simulink model "simu1"  (R2014b)
settings: Solver=VariableStepAuto  StartTime=0.0  StopTime=10.0  RelTol=1e-3
undefined symbols (not defined in the file or in its folder): As, Gamma1
libraries: simulink_extras x1
settings Model: Creator=e1302259  LastModifiedBy=Wissale !
settings DataIOCC: LimitDataPoints=off  SaveFormat=Dataset
settings OptimizationCC: UseDivisionForNetSlopeComputation=off  SimCompilerOptimization=off
settings DebuggingCC: SolverPrmCheckMsg=none  FrameProcessingCompatibilityMsg=error
settings HardwareCC: ProdBitPerPointer=64  ProdLargestAtomicFloat=Float  ProdIntDivRoundTo=Zero  ProdEndianess=LittleEndian  ProdWordSize=64  ProdHWDeviceType=Intel->x86-64 (Windows64)
settings ModelReferenceCC: PropagateSignalLabelsOutOfModel=on
settings RTWCC: RTWCompilerOptimization=off
settings ConfigComp: CovMetricSettings=dw  CovHtmlReporting=on  CovSaveCumulativeToWorkspaceVar=on  CovSaveSingleToWorkspaceVar=on  CovExternalEMLEnable=off

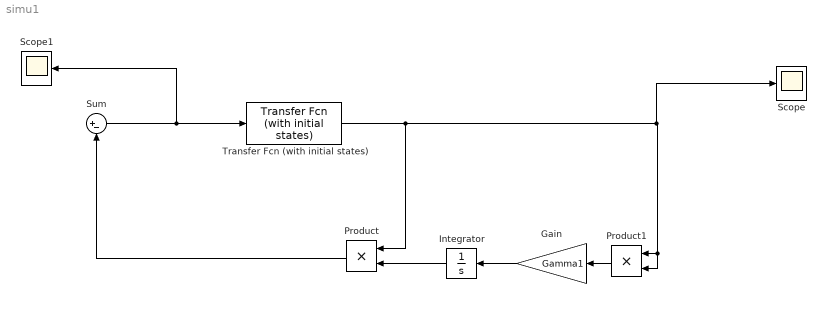
== system simu1 ==
  Gain : Gain  Gain=Gamma1
  Integrator : Integrator
  Product : Product
  Product1 : Product
  Scope : Scope
      settings: YMin=-0.57256  YMax=5.15304
  Scope1 : Scope
      settings: YMin=-0.57256  YMax=5.15304
  Sum : Sum  Inputs=|+-
  Transfer Fcn (with initial states) : simulink_extras/Additional Linear/Transfer Fcn (with initial states)  N=[1]  D="[1  As]"  X0=4
  wires:
  Transfer Fcn (with initial states)/1 -> Scope/1, Product1/2, Product1/1, Product/1
  Integrator/1 -> Product/2
  Gain/1 -> Integrator/1
  Product1/1 -> Gain/1
  Product/1 -> Sum/2
  Sum/1 -> Scope1/1, Transfer Fcn (with initial states)/1
